simulink library "DCMotorLibrary"  (R2020a)
settings: Solver=ode45  StartTime=0.0  StopTime=10.0  RelTol=1e-3
undefined symbols (not defined in the file or in its folder): b, deg, F, Fs, J, K, L, Motor, Motor_Lib, NULL, R, s, serial
libraries: fl_lib x69, nesl_utility x46, mblibv1 x13, ee_lib x12, sdl_lib x3, sm_lib x3, instrumentlib x3, simulink_extras x3, speedgoatlib_IO101 x3, simulink x1, $bdroot x1, demoLibrary x1
(part 1 of 2)
settings Model: Creator=deastman  LastModifiedBy=RAJENDRA PHUTANE
settings DataIOCC: LimitDataPoints=on  SaveFormat=Array  ReturnWorkspaceOutputs=off
settings OptimizationCC: BlockReduction=off  BooleanDataType=off  LifeSpan=inf
settings DebuggingCC: SaveWithParameterizedLinksMsg=none  UnderspecifiedInitializationDetection=Classic  MergeDetectMultiDrivingBlocksExec=none  SignalResolutionControl=TryResolveAllWithWarning  SFUnexpectedBacktrackingDiag=warning  SFNoUnconditionalDefaultTransitionDiag=warning  SFExecutionAtInitializationDiag=none  ArithmeticOperatorsInVariantConditions=warning
settings HardwareCC: ProdBitPerPointer=32  ProdBitPerSizeT=32  ProdBitPerPtrDiffT=32  ProdLargestAtomicFloat=None  ProdIntDivRoundTo=Undefined  ProdEndianess=Unspecified  ProdWordSize=32  ProdHWDeviceType=32-bit Generic  TargetUnknown=on
settings ModelReferenceCC: PropagateSignalLabelsOutOfModel=off
settings SFSimCC: SimUseLocalCustomCode=off  CustomCodeUndefinedFunction=UseInterfaceOnly
settings RTWCC: RTWUseLocalCustomCode=off
settings CodeAppCC: StateflowObjectComments=on
settings GRTTargetCC: TargetLangStandard=C89/C90 (ANSI)
settings ConfigComp: CovMetricSettings=dw  CovHtmlReporting=on  CovSaveCumulativeToWorkspaceVar=on  CovSaveSingleToWorkspaceVar=on  CovExternalEMLEnable=off  CovSFcnEnable=off

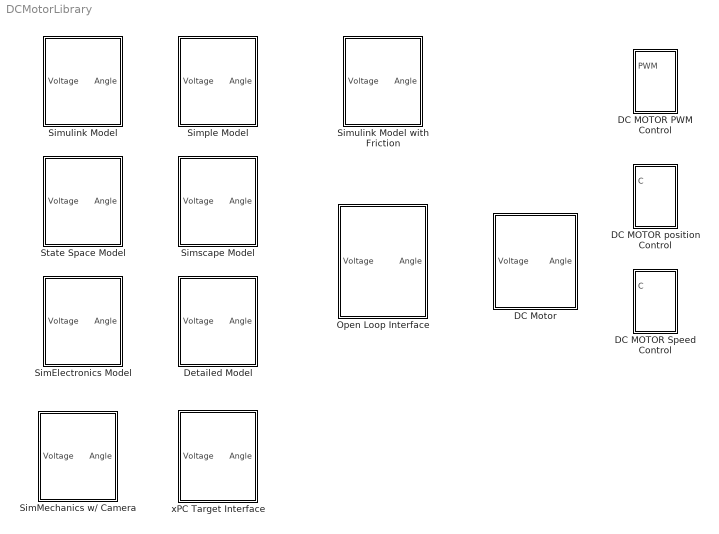
== system DCMotorLibrary ==
  DC MOTOR PWM Control : Subsystem
  DC MOTOR Speed Control : Subsystem
  DC MOTOR position Control : Subsystem
  DC Motor : Subsystem  BlockChoice=Open Loop Interface
      settings: TemplateBlock=self  MemberBlocks=Detailed Model,Open Loop Interface,SimElectronics Model,SimMechanics w/ Camera,Simple Model,Simscape Model,Simulink Model,Simulink Model with Friction,State Space Model,xPC Target Interface
  Detailed Model : Subsystem  mask(DC Motor){b=b, J=J, F=F, Fs=Fs, voltGain=1, Td=0.01}
      mask prompts: b "Damping Coefficient:"; J "Rotor Inertia:"; F "Friction:"; Fs "Staic Friction Gain:"; voltGain "Amplifier Gain:"; Td "Measurement Delay:"
      mask help:
      | This block simulates a basic brushed DC Motor with voltage input and rotor
      | angle in degrees as the output.
      mask Display: image(imread('dcmotor.jpg'))
  Open Loop Interface : Subsystem
      mask Display: image(imread('hs422.jpg'))
  SimElectronics Model : Subsystem  mask(DC Motor){K=K, R=R, L=L, b=b, J=J}
      mask prompts: K "Torque Constant:"; R "Armature Resistance:"; L "Armature Inductance:"; b "Damping Coefficient:"; J "Rotor Inertia:"
      mask help:
      | This block simulates a basic brushed DC Motor with voltage input and rotor
      | angle in degrees as the output.
      mask Display: image(imread('dcmotor.jpg'))
  SimMechanics w/ Camera : Subsystem  mask(DC Motor){K=K, R=R, L=L, b=b, J=J, Td=0.01}
      mask prompts: K "Torque Constant [N*m/A]"; R "Armature Resistance [Ohm]"; L "Armature Inductance [H]"; b "Damping Coefficient [N*m/(rad/s)]"; J "Rotor Inertia [g*cm^2]"; Td "Measurement Delay [s]"
      mask help:
      | This block simulates a basic brushed DC Motor with voltage input and rotor
      | angle in degrees as the output.
      mask Display: image(imread('dcmotor.jpg'))
  Simple Model : Subsystem  mask(DC Motor){K=K, F=F, Td=0}
      mask prompts: K "Motor Gain:"; F "Friction:"; Td "Time Delay:"
      mask help:
      | This block simulates a basic brushed DC Motor with voltage input and rotor
      | angle in degrees as the output.
      mask Display: image(imread('dcmotor.jpg'))
  Simscape Model : Subsystem  mask(DC Motor){K=K, R=R, L=L, b=b, J=J}
      mask prompts: K "Torque Constant:"; R "Armature Resistance:"; L "Armature Inductance:"; b "Damping Coefficient:"; J "Rotor Inertia:"
      mask help:
      | This block simulates a basic brushed DC Motor with voltage input and rotor
      | angle in degrees as the output.
      mask Display: image(imread('dcmotor.jpg'))
  Simulink Model : Subsystem  mask(DC Motor){K=K, R=R, L=L, b=b, J=J}
      mask prompts: K "Torque Constant:"; R "Armature Resistance:"; L "Armature Inductance:"; b "Damping Coefficient:"; J "Rotor Inertia:"
      mask help:
      | This block simulates a basic brushed DC Motor with voltage input and rotor
      | angle in degrees as the output.
      mask Display: image(imread('dcmotor.jpg'))
  Simulink Model with Friction : Subsystem  AncestorBlock=demoLibrary/Motor Models/Simulink Model  mask(DC Motor){K=K, R=R, L=L, F=F, Fs=Fs, J=J}
      mask prompts: K "Torque Constant:"; R "Armature Resistance:"; L "Armature Inductance:"; F "Coulomb Friction Torque:"; Fs "Static Friction Torque"; J "Rotor Inertia:"
      mask help:
      | This block simulates a basic brushed DC Motor with voltage input and rotor
      | angle in degrees as the output.
      mask Display: image(imread('dcmotor.jpg'))
  State Space Model : Subsystem  mask(DC Motor){K=K, R=R, L=L, b=b, J=J}
      mask prompts: K "Torque Constant:"; R "Armature Resistance:"; L "Armature Inductance:"; b "Damping Coefficient:"; J "Rotor Inertia:"
      mask help:
      | This block simulates a basic brushed DC Motor with voltage input and rotor
      | angle in degrees as the output.
      mask Display: image(imread('dcmotor.jpg'))
  xPC Target Interface : Subsystem
      mask Display: image(imread('xPCTargetDCMotor.jpg'))

== system DCMotorLibrary/DC MOTOR PWM Control ==
  PWM : Inport
  DC Source : fl_lib/Electrical/Electrical Sources/DC Voltage Source  v0=12 V
  ERef : fl_lib/Electrical/Electrical Elements/Electrical Reference
  Motor1 : Subsystem  VariantControl=Motor
      mask Display: image('youBot_Arm_Actuation_Motor_Motor_IMAGE.jpg');
  Scope : Scope
  Solver Configuration : nesl_utility/Solver Configuration  PhysicalDomain=network_engine_domain  SubClassName=solver  LeftPortType=input  RightPortType=generic  Tones=[]  Harmonics=[]  SimulateNoise=off  Profile=off  UseLocalSampling=off  EnableSwitchedLinearOptims=on  FrequencyDomain=off  UseCCode=off  RelTol=0.001  AbsTol=1e-06  MinStep=1e-09  ToWorkspace=off  RevertToSquareIcSolve=off  NumHomotopyIterations=100  PhasorMode=off  PhasorModeNumHarmonics=1  DoDC=off  ResidualTolerance=1e-09  UseLocalSolver=off  LocalSolverChoice=NE_BACKWARD_EULER_ADVANCER  LocalSolverSampleTime=0.001  DoFixedCost=off  MaxNonlinIter=3  MaxModeIter=2  LinearAlgebra=auto  EquationFormulation=NE_TIME_EF  DelaysMemoryBudget=1024  AutomaticFiltering=on  FilteringTimeConstant=0.001  PartitionStorageMethod=AS_NEEDED  PartitionMemoryBudget=1024  PartitionMethod=ROBUST
  F : PMIOPort  Side=Right
  B : PMIOPort  Port=2  Side=Left
  wires:
  Motor1/1(m) -> Scope/1
  PWM/1 -> Motor1/1(PWM)
  connections:
  DC Source/RConn1 -- Motor1/RConn2 -- ERef/LConn1
  DC Source/LConn1 -- Motor1/LConn2 -- Solver Configuration/RConn1
  Motor1/LConn1 -- B/RConn1
  Motor1/RConn1 -- F/RConn1

== system DCMotorLibrary/DC MOTOR Speed Control ==
  C : Inport
  DC Source : fl_lib/Electrical/Electrical Sources/DC Voltage Source  v0=12 V
  ERef : fl_lib/Electrical/Electrical Elements/Electrical Reference
  Motor1 : Subsystem  VariantControl=Motor
      mask Display: image('youBot_Arm_Actuation_Motor_Motor_IMAGE.jpg');
  Solver Configuration : nesl_utility/Solver Configuration  PhysicalDomain=network_engine_domain  SubClassName=solver  LeftPortType=input  RightPortType=generic  Tones=[]  Harmonics=[]  SimulateNoise=off  Profile=off  UseLocalSampling=off  EnableSwitchedLinearOptims=on  FrequencyDomain=off  UseCCode=off  RelTol=0.001  AbsTol=1e-06  MinStep=1e-09  ToWorkspace=off  RevertToSquareIcSolve=off  NumHomotopyIterations=100  PhasorMode=off  PhasorModeNumHarmonics=1  DoDC=off  ResidualTolerance=1e-09  UseLocalSolver=off  LocalSolverChoice=NE_BACKWARD_EULER_ADVANCER  LocalSolverSampleTime=0.001  DoFixedCost=off  MaxNonlinIter=3  MaxModeIter=2  LinearAlgebra=auto  EquationFormulation=NE_TIME_EF  DelaysMemoryBudget=1024  AutomaticFiltering=on  FilteringTimeConstant=0.001  PartitionStorageMethod=AS_NEEDED  PartitionMemoryBudget=1024  PartitionMethod=ROBUST
  Terminator : Terminator
  F : PMIOPort  Side=Right
  B : PMIOPort  Port=2  Side=Left
  wires:
  Motor1/1(m) -> Terminator/1
  C/1 -> Motor1/1(C)
  connections:
  DC Source/RConn1 -- Motor1/RConn2 -- ERef/LConn1
  DC Source/LConn1 -- Motor1/LConn2 -- Solver Configuration/RConn1
  Motor1/LConn1 -- B/RConn1
  Motor1/RConn1 -- F/RConn1

== system DCMotorLibrary/DC MOTOR position Control ==
  C : Inport
  DC Source : fl_lib/Electrical/Electrical Sources/DC Voltage Source  v0=12 V
  ERef : fl_lib/Electrical/Electrical Elements/Electrical Reference
  Motor1 : Subsystem  VariantControl=Motor
      mask Display: image('youBot_Arm_Actuation_Motor_Motor_IMAGE.jpg');
  Solver Configuration : nesl_utility/Solver Configuration  PhysicalDomain=network_engine_domain  SubClassName=solver  LeftPortType=input  RightPortType=generic  Tones=[]  Harmonics=[]  SimulateNoise=off  Profile=off  UseLocalSampling=off  EnableSwitchedLinearOptims=on  FrequencyDomain=off  UseCCode=off  RelTol=0.001  AbsTol=1e-06  MinStep=1e-09  ToWorkspace=off  RevertToSquareIcSolve=off  NumHomotopyIterations=100  PhasorMode=off  PhasorModeNumHarmonics=1  DoDC=off  ResidualTolerance=1e-09  UseLocalSolver=off  LocalSolverChoice=NE_BACKWARD_EULER_ADVANCER  LocalSolverSampleTime=0.001  DoFixedCost=off  MaxNonlinIter=3  MaxModeIter=2  LinearAlgebra=auto  EquationFormulation=NE_TIME_EF  DelaysMemoryBudget=1024  AutomaticFiltering=on  FilteringTimeConstant=0.001  PartitionStorageMethod=AS_NEEDED  PartitionMemoryBudget=1024  PartitionMethod=ROBUST
  Terminator : Terminator
  F : PMIOPort  Side=Right
  B : PMIOPort  Port=2  Side=Left
  wires:
  C/1 -> Motor1/1(C)
  Motor1/1(m) -> Terminator/1
  connections:
  Motor1/RConn1 -- F/RConn1
  Motor1/LConn1 -- B/RConn1
  Solver Configuration/RConn1 -- Motor1/LConn2 -- DC Source/LConn1
  ERef/LConn1 -- Motor1/RConn2 -- DC Source/RConn1

== system DCMotorLibrary/DC Motor ==
  Voltage : Inport
  Open Loop Interface : $bdroot/Motor Models/Open Loop Interface  SystemSampleTime=-1  Latency=0  AutoFrameSizeCalculation=off
  Angle : Outport
  wires:
  Voltage/1 -> Open Loop Interface/1
  Open Loop Interface/1 -> Angle/1

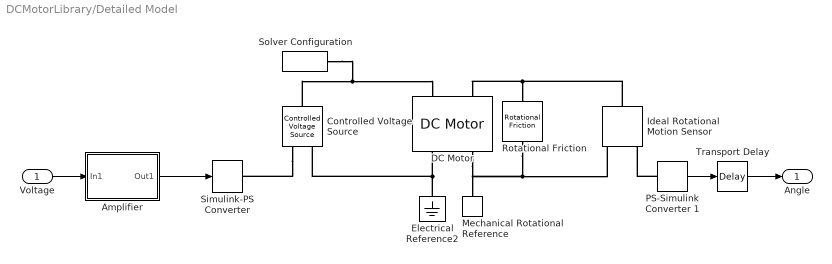
== system DCMotorLibrary/Detailed Model ==
  Voltage : Inport
  Amplifier : Subsystem
  Controlled Voltage Source : fl_lib/Electrical/Electrical Sources/Controlled Voltage Source
  DC Motor : ee_lib/Electromechanical/Brushed Motors/DC Motor  field_option=ee.enum.field_option.pm  Rf=100 Ohm  Lf=1 H  Laf=0.15 H  If0=0 A  parameterization=2  Ra=8 Ohm  La=1.5e-3 H  emf_or_torque=1  Kv=1 V/(rad/s)  Ki=6.876e-04 N*m/A  T_stall=57/16 in*lbf  w_max=62.5 rpm  w_rated=1.5e+04 rpm  P_rated=0.08 W  V_rated=5 V  J=J kg*m^2  lam_param=1  lam=b N*m/(rad/s)  i_noload=0 A  V_i_noload=1.5 V  speed0=0 rpm  alpha=3.93e-3 1/K  Tmeas=25 degC  thermal_mass=100 J/K  initial_temperature=25 degC
  Electrical Reference2 : fl_lib/Electrical/Electrical Elements/Electrical Reference
  Ideal Rotational Motion Sensor : fl_lib/Mechanical/Mechanical Sensors/Ideal Rotational Motion Sensor  wrap_angle=simscape.enum.onoff.off  offset=0 rad
  Mechanical Rotational Reference : fl_lib/Mechanical/Rotational Elements/Mechanical Rotational Reference
  PS-Simulink Converter 1 : nesl_utility/PS-Simulink Converter  PhysicalDomain=network_engine_domain  SubClassName=ps_output  LeftPortType=input  RightPortType=output  PseudoPeriodic=off  Frequencies=[]  Unit=deg  AffineConversion=off
  Rotational Friction : fl_lib/Mechanical/Rotational Elements/Rotational Friction  brkwy_trq=F*Fs N*m  brkwy_vel=0.060623 rad/s  Col_trq=F N*m  visc_coef=0.001 N*m/(rad/s)  w_specify=off  w_priority=High  w=0 rad/s  w_nominal_specify=off  w_nominal_unit=rad/s  w_nominal_value=1  t_specify=off  t_priority=High  t=0 N*m  t_nominal_specify=off  t_nominal_unit=N*m  t_nominal_value=1
  Simulink-PS Converter : nesl_utility/Simulink-PS Converter  PhysicalDomain=network_engine_domain  SubClassName=ps_input  LeftPortType=input  RightPortType=output  PseudoPeriodic=off  Frequencies=[]  NoiseDistribution=none  NoiseParameters=[]  Unit=1  AffineConversion=off  FilteringAndDerivatives=zero  SimscapeFilterOrder=1  InputFilterTimeConstant=.001  UdotUserProvided=0
  Solver Configuration : nesl_utility/Solver Configuration  PhysicalDomain=network_engine_domain  SubClassName=solver  LeftPortType=input  RightPortType=generic  Tones=[]  Harmonics=[]  SimulateNoise=off  Profile=off  UseLocalSampling=off  EnableSwitchedLinearOptims=on  FrequencyDomain=off  UseCCode=off  RelTol=0.001  AbsTol=1e-06  MinStep=1e-09  ToWorkspace=off  RevertToSquareIcSolve=off  NumHomotopyIterations=100  PhasorMode=off  PhasorModeNumHarmonics=1  DoDC=off  ResidualTolerance=1e-9  UseLocalSolver=off  LocalSolverChoice=NE_BACKWARD_EULER_ADVANCER  LocalSolverSampleTime=.001  DoFixedCost=off  MaxNonlinIter=12  MaxModeIter=2  LinearAlgebra=Sparse  EquationFormulation=NE_TIME_EF  DelaysMemoryBudget=1024  AutomaticFiltering=on  FilteringTimeConstant=0.001  PartitionStorageMethod=AS_NEEDED  PartitionMemoryBudget=1024  PartitionMethod=FAST
  Transport Delay : TransportDelay  DelayTime=Td  PadeOrder=4
  Angle : Outport
  wires:
  Voltage/1 -> Amplifier/1(In1)
  PS-Simulink Converter 1/1 -> Transport Delay/1
  Transport Delay/1 -> Angle/1
  Amplifier/1(Out1) -> Simulink-PS Converter/1
  connections:
  Ideal Rotational Motion Sensor/LConn1 -- DC Motor/LConn2 -- Rotational Friction/LConn1
  Controlled Voltage Source/RConn1 -- Simulink-PS Converter/RConn1
  PS-Simulink Converter 1/LConn1 -- Ideal Rotational Motion Sensor/RConn3
  Mechanical Rotational Reference/LConn1 -- DC Motor/RConn2 -- Ideal Rotational Motion Sensor/RConn1 -- Rotational Friction/RConn1
  Controlled Voltage Source/LConn1 -- DC Motor/LConn1 -- Solver Configuration/RConn1
  Electrical Reference2/LConn1 -- DC Motor/RConn1 -- Controlled Voltage Source/RConn2

== system DCMotorLibrary/Open Loop Interface ==
  Voltage : Inport
  Bias : Bias  Bias=5
  Gain : Gain  Gain=255/10  OutDataTypeStr=uint8
  Saturation1 : Saturate  UpperLimit=5  LowerLimit=-5
  Serial Motor Interface : Subsystem  AncestorBlock=demoLibrary/Utilities/Serial Motor Interface
  Simulation Pace : aerolibanimutils/Simulation Pace  SimulationPace=1  SleepMode=MATLAB Thread  OutputPaceError=off  SampleTime=1/50
      settings: AttributesFormatString=%<SimulationPace> sec/sec
  Angle : Outport  PortDimensions=1
  wires:
  Voltage/1 -> Saturation1/1
  Serial Motor Interface/1(Angle) -> Angle/1
  Saturation1/1 -> Bias/1
  Bias/1 -> Gain/1
  Gain/1 -> Serial Motor Interface/1(command)

== system DCMotorLibrary/SimElectronics Model ==
  Voltage : Inport
  Controlled Voltage Source : fl_lib/Electrical/Electrical Sources/Controlled Voltage Source
  DC Motor : ee_lib/Electromechanical/Brushed Motors/DC Motor  field_option=ee.enum.field_option.pm  Rf=100 Ohm  Lf=1 H  Laf=0.15 H  If0=0 A  parameterization=1  Ra=R Ohm  La=L H  emf_or_torque=1  Kv=K V/(rad/s)  Ki=6.876e-04 N*m/A  T_stall=2.4e-04 N*m  w_max=1.91e+04 rpm  w_rated=1.5e+04 rpm  P_rated=0.08 W  V_rated=1.5 V  J=J kg*m^2  lam_param=1  lam=b N*m/(rad/s)  i_noload=0 A  V_i_noload=1.5 V  speed0=0 rpm  alpha=3.93e-3 1/K  Tmeas=25 degC  thermal_mass=100 J/K  initial_temperature=25 degC
  Electrical Reference2 : fl_lib/Electrical/Electrical Elements/Electrical Reference
  Ideal Rotational Motion Sensor : fl_lib/Mechanical/Mechanical Sensors/Ideal Rotational Motion Sensor  wrap_angle=simscape.enum.onoff.off  offset=0 rad
  Mechanical Rotational Reference : fl_lib/Mechanical/Rotational Elements/Mechanical Rotational Reference
  PS-Simulink Converter 1 : nesl_utility/PS-Simulink Converter  PhysicalDomain=network_engine_domain  SubClassName=ps_output  LeftPortType=input  RightPortType=output  PseudoPeriodic=off  Frequencies=[]  Unit=deg  AffineConversion=off
  Simulink-PS Converter : nesl_utility/Simulink-PS Converter  PhysicalDomain=network_engine_domain  SubClassName=ps_input  LeftPortType=input  RightPortType=output  PseudoPeriodic=off  Frequencies=[]  NoiseDistribution=none  NoiseParameters=[]  Unit=1  AffineConversion=off  FilteringAndDerivatives=zero  SimscapeFilterOrder=1  InputFilterTimeConstant=.001  UdotUserProvided=0
  Solver Configuration : nesl_utility/Solver Configuration  PhysicalDomain=network_engine_domain  SubClassName=solver  LeftPortType=input  RightPortType=generic  Tones=[]  Harmonics=[]  SimulateNoise=off  Profile=off  UseLocalSampling=off  EnableSwitchedLinearOptims=on  FrequencyDomain=off  UseCCode=off  RelTol=0.001  AbsTol=1e-06  MinStep=1e-09  ToWorkspace=off  RevertToSquareIcSolve=off  NumHomotopyIterations=100  PhasorMode=off  PhasorModeNumHarmonics=1  DoDC=off  ResidualTolerance=1e-9  UseLocalSolver=off  LocalSolverChoice=NE_BACKWARD_EULER_ADVANCER  LocalSolverSampleTime=.001  DoFixedCost=off  MaxNonlinIter=3  MaxModeIter=2  LinearAlgebra=Sparse  EquationFormulation=NE_TIME_EF  DelaysMemoryBudget=1024  AutomaticFiltering=on  FilteringTimeConstant=0.001  PartitionStorageMethod=AS_NEEDED  PartitionMemoryBudget=1024  PartitionMethod=FAST
  Angle : Outport
  wires:
  PS-Simulink Converter 1/1 -> Angle/1
  Voltage/1 -> Simulink-PS Converter/1
  connections:
  DC Motor/LConn1 -- Solver Configuration/RConn1 -- Controlled Voltage Source/LConn1
  DC Motor/RConn1 -- Controlled Voltage Source/RConn2 -- Electrical Reference2/LConn1
  DC Motor/RConn2 -- Ideal Rotational Motion Sensor/RConn1 -- Mechanical Rotational Reference/LConn1
  PS-Simulink Converter 1/LConn1 -- Ideal Rotational Motion Sensor/RConn3
  Controlled Voltage Source/RConn1 -- Simulink-PS Converter/RConn1
  Ideal Rotational Motion Sensor/LConn1 -- DC Motor/LConn2

== system DCMotorLibrary/SimMechanics w// Camera ==
  Voltage : Inport
  Controlled Voltage Source : fl_lib/Electrical/Electrical Sources/Controlled Voltage Source
  DC Motor : ee_lib/Electromechanical/Brushed Motors/DC Motor  field_option=ee.enum.field_option.pm  Rf=100 Ohm  Lf=1 H  Laf=0.15 H  If0=0 A  parameterization=1  Ra=R Ohm  La=L H  emf_or_torque=2  Kv=7.2e-05 V/rpm  Ki=K N*m/A  T_stall=2.4e-04 N*m  w_max=1.91e+04 rpm  w_rated=1.5e+04 rpm  P_rated=0.08 W  V_rated=1.5 V  J=J g*cm^2  lam_param=1  lam=b N*m/(rad/s)  i_noload=0 A  V_i_noload=1.5 V  speed0=0 rpm  alpha=3.93e-3 1/K  Tmeas=25 degC  thermal_mass=100 J/K  initial_temperature=25 degC
  Electrical Reference : fl_lib/Electrical/Electrical Elements/Electrical Reference
  Mechanical Rotational Reference : fl_lib/Mechanical/Rotational Elements/Mechanical Rotational Reference
  Mechanical part : Subsystem
      mask Display: image(imread('hs422.jpg'))
  Revolute - Rotational Interface : mblibv1/Interface  Elements/Revolute - Rotational Interface  UpdateFromCAD=off  DialogClass=RevoluteRotationalInterface  Primitive=R1  InputFiltering=off  SimscapeFilterOrder=1  InputFilterTimeConstant=0.001
  Simulink-PS Converter : nesl_utility/Simulink-PS Converter  PhysicalDomain=network_engine_domain  SubClassName=ps_input  LeftPortType=input  RightPortType=output  PseudoPeriodic=off  Frequencies=[]  NoiseDistribution=none  NoiseParameters=[]  Unit=1  AffineConversion=off  FilteringAndDerivatives=filter  SimscapeFilterOrder=2  InputFilterTimeConstant=.001  UdotUserProvided=1
  Solver Configuration : nesl_utility/Solver Configuration  PhysicalDomain=network_engine_domain  SubClassName=solver  LeftPortType=input  RightPortType=generic  Tones=[]  Harmonics=[]  SimulateNoise=off  Profile=off  UseLocalSampling=off  EnableSwitchedLinearOptims=on  FrequencyDomain=off  UseCCode=off  RelTol=0.001  AbsTol=1e-06  MinStep=1e-09  ToWorkspace=off  RevertToSquareIcSolve=off  NumHomotopyIterations=100  PhasorMode=off  PhasorModeNumHarmonics=1  DoDC=off  ResidualTolerance=1e-9  UseLocalSolver=on  LocalSolverChoice=NE_BACKWARD_EULER_ADVANCER  LocalSolverSampleTime=.001  DoFixedCost=off  MaxNonlinIter=12  MaxModeIter=2  LinearAlgebra=Sparse  EquationFormulation=NE_TIME_EF  DelaysMemoryBudget=1024  AutomaticFiltering=on  FilteringTimeConstant=0.001  PartitionStorageMethod=AS_NEEDED  PartitionMemoryBudget=1024  PartitionMethod=FAST
  Transport Delay : TransportDelay  DelayTime=Td  PadeOrder=4
  Angle : Outport
  wires:
  Transport Delay/1 -> Angle/1
  Mechanical part/1(Angle) -> Transport Delay/1
  Voltage/1 -> Simulink-PS Converter/1
  connections:
  Revolute - Rotational Interface/RConn1 -- Mechanical part/LConn1
  DC Motor/LConn2 -- Revolute - Rotational Interface/LConn1
  Simulink-PS Converter/RConn1 -- Controlled Voltage Source/RConn1
  Mechanical Rotational Reference/LConn1 -- Revolute - Rotational Interface/LConn2 -- DC Motor/RConn2
  Solver Configuration/RConn1 -- Controlled Voltage Source/LConn1 -- DC Motor/LConn1
  Controlled Voltage Source/RConn2 -- DC Motor/RConn1 -- Electrical Reference/LConn1

== system DCMotorLibrary/Simple Model ==
  Voltage : Inport
  Dead Zone : DeadZone  LowerValue=-F  UpperValue=F  SaturateOnIntegerOverflow=on
  Gain : Gain  Gain=K
  Integrator : Integrator
  Transport Delay : TransportDelay  DelayTime=Td  PadeOrder=4
  Angle : Outport
  wires:
  Dead Zone/1 -> Gain/1
  Voltage/1 -> Dead Zone/1
  Integrator/1 -> Transport Delay/1
  Gain/1 -> Integrator/1
  Transport Delay/1 -> Angle/1

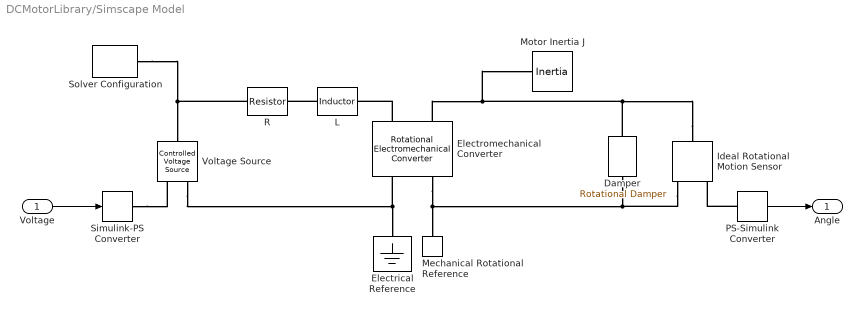
== system DCMotorLibrary/Simscape Model ==
  Voltage : Inport
  Damper : fl_lib/Mechanical/Rotational Elements/Rotational Damper  D=b N*m/(rad/s)  w_specify=off  w_priority=None  w=0 rad/s  w_nominal_specify=off  w_nominal_unit=rad/s  w_nominal_value=1  t_specify=off  t_priority=None  t=0 N*m  t_nominal_specify=off  t_nominal_unit=N*m  t_nominal_value=1
  Electrical Reference : fl_lib/Electrical/Electrical Elements/Electrical Reference
  Electromechanical Converter : fl_lib/Electrical/Electrical Elements/Rotational Electromechanical Converter  K=K V/(rad/s)  i_specify=off  i_priority=None  i=0 A  i_nominal_specify=off  i_nominal_unit=A  i_nominal_value=1  v_specify=off  v_priority=None  v=0 V  v_nominal_specify=off  v_nominal_unit=V  v_nominal_value=1  t_specify=off  t_priority=None  t=0 N*m  t_nominal_specify=off  t_nominal_unit=N*m  t_nominal_value=1  w_specify=off  w_priority=None  w=0 rad/s  w_nominal_specify=off  w_nominal_unit=rad/s  w_nominal_value=1
  Ideal Rotational Motion Sensor : fl_lib/Mechanical/Mechanical Sensors/Ideal Rotational Motion Sensor  wrap_angle=simscape.enum.onoff.off  offset=0 deg
  L : fl_lib/Electrical/Electrical Elements/Inductor  l=L H  r=0 Ohm  g=1e-09 1/Ohm  i_specify=off  i_priority=None  i=0 A  i_nominal_specify=off  i_nominal_unit=A  i_nominal_value=1  v_specify=off  v_priority=None  v=0 V  v_nominal_specify=off  v_nominal_unit=V  v_nominal_value=1  i_L_specify=on  i_L_priority=High  i_L=0 A  i_L_nominal_specify=off  i_L_nominal_unit=A  i_L_nominal_value=1
  Mechanical Rotational Reference : fl_lib/Mechanical/Rotational Elements/Mechanical Rotational Reference
  Motor Inertia J : fl_lib/Mechanical/Rotational Elements/Inertia  inertia=J kg*m^2  w_specify=on  w_priority=High  w=0 rad/s  w_nominal_specify=off  w_nominal_unit=rad/s  w_nominal_value=1  t_specify=off  t_priority=None  t=0 N*m  t_nominal_specify=off  t_nominal_unit=N*m  t_nominal_value=1
  PS-Simulink Converter : nesl_utility/PS-Simulink Converter  PhysicalDomain=network_engine_domain  SubClassName=ps_output  LeftPortType=input  RightPortType=output  PseudoPeriodic=off  Frequencies=[]  Unit=deg  AffineConversion=off
  R : fl_lib/Electrical/Electrical Elements/Resistor  Tag=Factory Generic  R=R Ohm  i_specify=off  i_priority=None  i=0 A  i_nominal_specify=off  i_nominal_unit=A  i_nominal_value=1  v_specify=off  v_priority=None  v=0 V  v_nominal_specify=off  v_nominal_unit=V  v_nominal_value=1
  Simulink-PS Converter : nesl_utility/Simulink-PS Converter  PhysicalDomain=network_engine_domain  SubClassName=ps_input  LeftPortType=input  RightPortType=output  PseudoPeriodic=off  Frequencies=[]  NoiseDistribution=none  NoiseParameters=[]  Unit=V  AffineConversion=off  FilteringAndDerivatives=zero  SimscapeFilterOrder=1  InputFilterTimeConstant=.001  UdotUserProvided=0
  Solver Configuration : nesl_utility/Solver Configuration  PhysicalDomain=network_engine_domain  SubClassName=solver  LeftPortType=input  RightPortType=generic  Tones=[]  Harmonics=[]  SimulateNoise=off  Profile=off  UseLocalSampling=off  EnableSwitchedLinearOptims=on  FrequencyDomain=off  UseCCode=off  RelTol=0.001  AbsTol=1e-06  MinStep=1e-09  ToWorkspace=off  RevertToSquareIcSolve=off  NumHomotopyIterations=100  PhasorMode=off  PhasorModeNumHarmonics=1  DoDC=off  ResidualTolerance=1e-9  UseLocalSolver=off  LocalSolverChoice=NE_BACKWARD_EULER_ADVANCER  LocalSolverSampleTime=.001  DoFixedCost=off  MaxNonlinIter=3  MaxModeIter=2  LinearAlgebra=Sparse  EquationFormulation=NE_TIME_EF  DelaysMemoryBudget=1024  AutomaticFiltering=on  FilteringTimeConstant=0.001  PartitionStorageMethod=AS_NEEDED  PartitionMemoryBudget=1024  PartitionMethod=FAST
  Voltage Source : fl_lib/Electrical/Electrical Sources/Controlled Voltage Source
  Angle : Outport
  wires:
  Voltage/1 -> Simulink-PS Converter/1
  PS-Simulink Converter/1 -> Angle/1
  connections:
  R/LConn1 -- Solver Configuration/RConn1 -- Voltage Source/LConn1
  Electromechanical Converter/RConn1 -- Voltage Source/RConn2 -- Electrical Reference/LConn1
  Ideal Rotational Motion Sensor/LConn1 -- Electromechanical Converter/LConn2 -- Motor Inertia J/LConn1 -- Damper/LConn1
  Ideal Rotational Motion Sensor/RConn1 -- Damper/RConn1 -- Mechanical Rotational Reference/LConn1 -- Electromechanical Converter/RConn2
  Simulink-PS Converter/RConn1 -- Voltage Source/RConn1
  Electromechanical Converter/LConn1 -- L/RConn1
  L/LConn1 -- R/RConn1
  PS-Simulink Converter/LConn1 -- Ideal Rotational Motion Sensor/RConn3

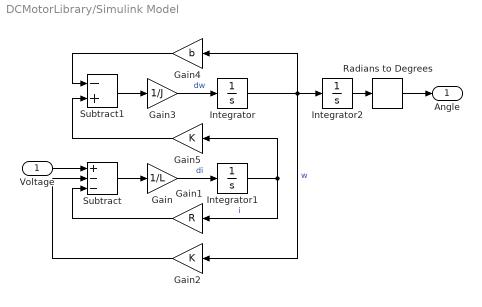
== system DCMotorLibrary/Simulink Model ==
  Voltage : Inport
  Gain : Gain  Gain=1/L
  Gain1 : Gain  Gain=R
  Gain2 : Gain  Gain=K
  Gain3 : Gain  Gain=1/J
  Gain4 : Gain  Gain=b
  Gain5 : Gain  Gain=K
  Integrator : Integrator
  Integrator1 : Integrator
  Integrator2 : Integrator
  Radians to Degrees : simulink_extras/Transformations/Radians to Degrees
  Subtract : Sum  Inputs=+--
  Subtract1 : Sum  Inputs=-+
  Angle : Outport
  wires:
  Voltage/1 -> Subtract/1
  Integrator2/1 -> Radians to Degrees/1
  Gain5/1 -> Subtract1/2
  Gain4/1 -> Subtract1/1
  Subtract1/1 -> Gain3/1
  Gain2/1 -> Subtract/2
  Gain1/1 -> Subtract/3
  Subtract/1 -> Gain/1
  Integrator1/1 -> Gain1/1, Gain5/1  "i"
  Integrator/1 -> Integrator2/1, Gain2/1, Gain4/1  "w"
  Gain/1 -> Integrator1/1  "di"
  Gain3/1 -> Integrator/1  "dw"
  Radians to Degrees/1 -> Angle/1

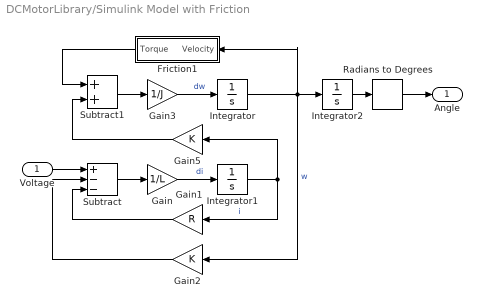
== system DCMotorLibrary/Simulink Model with Friction ==
  Voltage : Inport
  Friction1 : Subsystem  mask{FrictionStatic=Fs, FrictionCoulomb=F, eps=0.005}
      mask prompts: FrictionStatic "Static Friction Torque (Nm)"; FrictionCoulomb "Coulomb Friction Torque (Nm)"; eps "Epsilon (deg/s)"
  Gain : Gain  Gain=1/L
  Gain1 : Gain  Gain=R
  Gain2 : Gain  Gain=K
  Gain3 : Gain  Gain=1/J
  Gain5 : Gain  Gain=K
  Integrator : Integrator
  Integrator1 : Integrator
  Integrator2 : Integrator
  Radians to Degrees : simulink_extras/Transformations/Radians to Degrees
  Subtract : Sum  Inputs=+--
  Subtract1 : Sum
  Angle : Outport
  wires:
  Radians to Degrees/1 -> Angle/1
  Gain3/1 -> Integrator/1  "dw"
  Gain/1 -> Integrator1/1  "di"
  Integrator/1 -> Gain2/1, Friction1/1(Velocity), Integrator2/1  "w"
  Integrator1/1 -> Gain5/1, Gain1/1  "i"
  Subtract/1 -> Gain/1
  Gain1/1 -> Subtract/3
  Gain2/1 -> Subtract/2
  Subtract1/1 -> Gain3/1
  Gain5/1 -> Subtract1/2
  Integrator2/1 -> Radians to Degrees/1
  Voltage/1 -> Subtract/1
  Friction1/1(Torque) -> Subtract1/1

== system DCMotorLibrary/State Space Model ==
  Voltage : Inport
  Integrator2 : Integrator
  Radians to Degrees : simulink_extras/Transformations/Radians to Degrees
  State-Space : StateSpace  A=[-b/J K/J; -K/L -R/L]  B=[0; 1/L]  C=[1 0]  D=[0]  InitialCondition=0
  Angle : Outport
  wires:
  Integrator2/1 -> Radians to Degrees/1
  Voltage/1 -> State-Space/1
  State-Space/1 -> Integrator2/1
  Radians to Degrees/1 -> Angle/1

== system DCMotorLibrary/xPC Target Interface ==
  Voltage : Inport
  Analog input : speedgoatlib_IO101/Analog input  id=1  startChannel=2  numChannels=1  coupling=2  range=3  acqMode=1  outpMode=Values  ts=0.002  pciSlot=-1
  Digital output : speedgoatlib_IO101/Digital output  id=1  groupChannel=Upper  lowerChannel=1  upperChannel=[1,5,6]  lowerDOReset=1  upperDOReset=[0,0,0]  lowerDOInitValues=0  upperDOInitValues=[0,0,0]  ts=0.002  pciSlot=-1
  Setup : speedgoatlib_IO101/Setup  group=Digital setup upper channel  id=1  pciSlot=-1  adStartChannel=2  adNumChannel=1  adCoupling=Single-ended  adRange="-3.3 .. 3.3V ==> Set  hardware DIP switches 2 4 6 9 to ON"  adAcqMode=Standard  daChannel=[1:8]  daReset=[1]  daInitValue=[0]  lowerChannel=1  lowerDirection=Input  lowerDIDebounce=0  lowerDOReset=[1]  lowerDOInitValues=[0]  upperChannel=[1 5 6]  upperDirection=Output  upperDIDebounce=0  upperDOReset=0  upperDOInitValues=0
  SignalConditioning : SAM_lib/SignalConditioning
  Angle : Outport
  wires:
  SignalConditioning/3 -> Digital output/3
  Analog input/1 -> SignalConditioning/2
  SignalConditioning/4 -> Angle/1  "measured angle"
  Voltage/1 -> SignalConditioning/1
  SignalConditioning/1 -> Digital output/1
  SignalConditioning/2 -> Digital output/2

== system DCMotorLibrary/DC MOTOR PWM Control/Motor1 ==
  PWM : Inport
  Meas P : Subsystem  Tag=CustomStyle
      mask Display: disp('m')
  Motor : Subsystem  AncestorBlock=Motor_Lib/Motor  VariantControl=Motor  mask{r_motor=Motor.R, l_motor=Motor.L, k_motor=Motor.K, i_motor_noLoad=Motor.no_load_i, v_supply=Motor.V, gear_ratio=Motor.gr, friction_visc=Motor.friction, ctrl_deadZone=Motor.Dead_Band}
      mask prompts: r_motor "Armature Resistance (Ohm)"; l_motor "Armature Inductance (H)"; k_motor "Torque Constant (N*(m/A))"; i_motor_noLoad "No-Load Current (A)"; v_supply "Supply Voltage (V)"; gear_ratio "Gear Ratio"; friction_visc "Viscous Friction (N*m/(rad/s))"; ctrl_deadZone "Dead Zone (deg)"
      mask DialogControl Container4 Prompt: Electrical
      mask DialogControl Container5 Prompt: Mechanical
      mask DialogControl Container6 Prompt: Control
      mask Display: image('youBot_Arm_Motor_JointIntf_IMAGE.jpg');
  RevolutePivotBicep : sm_lib/Joints/Revolute Joint  JointMode=Normal  SenseConstraintForce=on  SenseConstraintForceX=off  SenseConstraintForceY=off  SenseConstraintForceZ=off  SenseConstraintTorque=off  SenseConstraintTorqueX=off  SenseConstraintTorqueY=off  SenseConstraintTorqueZ=off  SenseTotalForce=off  SenseTotalForceX=off  SenseTotalForceY=off  SenseTotalForceZ=off  SenseTotalTorque=off  SenseTotalTorqueX=off  SenseTotalTorqueY=off  SenseTotalTorqueZ=off  CompositeWrenchDir=FollowerOnBase  CompositeWrenchFrame=BaseFrame  EquilibriumPosition=0  EquilibriumPositionUnits=rad  SpringStiffness=0  SpringStiffnessUnits=N*m/rad  DampingCoefficient=0  DampingCoefficientUnits=N*m/(rad/s)  TorqueActuationMode=InputTorque  MotionActuationMode=ComputedMotion  SensePosition=on  SenseVelocity=on  SenseAcceleration=off  SenseTorqueForce=on  SenseLowerLimitTorqueForce=off  SenseUpperLimitTorqueForce=off  LowerLimitSpecify=off  LowerLimitBound=-90  LowerLimitBoundUnits=deg  LowerLimitStiffness=1e4  LowerLimitStiffnessUnits=N*m/deg  LowerLimitDamping=10  LowerLimitDampingUnits=N*m/(deg/s)  LowerLimitTransitionRegionWidth=0.1  LowerLimitTransitionRegionWidthUnits=deg  UpperLimitSpecify=off  UpperLimitBound=90  UpperLimitBoundUnits=deg  UpperLimitStiffness=1e4  UpperLimitStiffnessUnits=N*m/deg  UpperLimitDamping=10  UpperLimitDampingUnits=N*m/(deg/s)  UpperLimitTransitionRegionWidth=0.1  UpperLimitTransitionRegionWidthUnits=deg  PositionTargetSpecify=on  PositionTargetPriority=Low  PositionTargetValue=0  PositionTargetValueUnits=deg  VelocityTargetSpecify=off  VelocityTargetPriority=High  VelocityTargetValue=0  VelocityTargetValueUnits=deg/s
  Sensing i : Subsystem
      mask Display: disp('i')
  B : PMIOPort  Side=Left
  F : PMIOPort  Port=2  Side=Right
  - : PMIOPort  Port=3  Side=Right
  + : PMIOPort  Port=4  Side=Left
  m : Outport  VectorParamsAs1DForOutWhenUnconnected=off
  wires:
  Meas P/1(P) -> m/1
  PWM/1 -> Motor/1(PWM)
  connections:
  RevolutePivotBicep/RConn2 -- Meas P/LConn1
  Meas P/LConn3 -- RevolutePivotBicep/RConn4
  Meas P/LConn2 -- RevolutePivotBicep/RConn3 -- Motor/RConn1
  Motor/LConn1 -- RevolutePivotBicep/LConn2
  RevolutePivotBicep/RConn1 -- F/RConn1
  RevolutePivotBicep/LConn1 -- B/RConn1
  Sensing i/LConn1 -- Motor/RConn2
  Motor/LConn2 -- +/RConn1
  Sensing i/RConn2 -- -/RConn1
  Sensing i/RConn1 -- Meas P/LConn5
  RevolutePivotBicep/RConn5 -- Meas P/LConn4

== system DCMotorLibrary/DC MOTOR Speed Control/Motor1 ==
  C : Inport
  Meas P : Subsystem  Tag=CustomStyle
      mask Display: disp('m')
  Motor : Subsystem  AncestorBlock=Motor_Lib/Motor  VariantControl=Motor  mask{r_motor=Motor.R, l_motor=Motor.L, k_motor=Motor.K, i_motor_noLoad=Motor.no_load_i, v_supply=Motor.V, gear_ratio=Motor.gr, friction_visc=Motor.friction, ctrl_deadZone=Motor.Dead_Band}
      mask prompts: r_motor "Armature Resistance (Ohm)"; l_motor "Armature Inductance (H)"; k_motor "Torque Constant (N*(m/A))"; i_motor_noLoad "No-Load Current (A)"; v_supply "Supply Voltage (V)"; gear_ratio "Gear Ratio"; friction_visc "Viscous Friction (N*m/(rad/s))"; ctrl_deadZone "Dead Zone (deg)"
      mask DialogControl Container4 Prompt: Electrical
      mask DialogControl Container5 Prompt: Mechanical
      mask DialogControl Container6 Prompt: Control
      mask Display: image('youBot_Arm_Motor_JointIntf_IMAGE.jpg');
  RevolutePivotBicep : sm_lib/Joints/Revolute Joint  JointMode=Normal  SenseConstraintForce=on  SenseConstraintForceX=off  SenseConstraintForceY=off  SenseConstraintForceZ=off  SenseConstraintTorque=off  SenseConstraintTorqueX=off  SenseConstraintTorqueY=off  SenseConstraintTorqueZ=off  SenseTotalForce=off  SenseTotalForceX=off  SenseTotalForceY=off  SenseTotalForceZ=off  SenseTotalTorque=off  SenseTotalTorqueX=off  SenseTotalTorqueY=off  SenseTotalTorqueZ=off  CompositeWrenchDir=FollowerOnBase  CompositeWrenchFrame=BaseFrame  EquilibriumPosition=0  EquilibriumPositionUnits=rad  SpringStiffness=0  SpringStiffnessUnits=N*m/rad  DampingCoefficient=0  DampingCoefficientUnits=N*m/(rad/s)  TorqueActuationMode=InputTorque  MotionActuationMode=ComputedMotion  SensePosition=on  SenseVelocity=on  SenseAcceleration=off  SenseTorqueForce=on  SenseLowerLimitTorqueForce=off  SenseUpperLimitTorqueForce=off  LowerLimitSpecify=off  LowerLimitBound=-90  LowerLimitBoundUnits=deg  LowerLimitStiffness=1e4  LowerLimitStiffnessUnits=N*m/deg  LowerLimitDamping=10  LowerLimitDampingUnits=N*m/(deg/s)  LowerLimitTransitionRegionWidth=0.1  LowerLimitTransitionRegionWidthUnits=deg  UpperLimitSpecify=off  UpperLimitBound=90  UpperLimitBoundUnits=deg  UpperLimitStiffness=1e4  UpperLimitStiffnessUnits=N*m/deg  UpperLimitDamping=10  UpperLimitDampingUnits=N*m/(deg/s)  UpperLimitTransitionRegionWidth=0.1  UpperLimitTransitionRegionWidthUnits=deg  PositionTargetSpecify=on  PositionTargetPriority=Low  PositionTargetValue=0  PositionTargetValueUnits=deg  VelocityTargetSpecify=off  VelocityTargetPriority=High  VelocityTargetValue=0  VelocityTargetValueUnits=deg/s
  Sensing i : Subsystem
      mask Display: disp('i')
  B : PMIOPort  Side=Left
  F : PMIOPort  Port=2  Side=Right
  - : PMIOPort  Port=3  Side=Right
  + : PMIOPort  Port=4  Side=Left
  m : Outport  VectorParamsAs1DForOutWhenUnconnected=off
  wires:
  Meas P/1(P) -> m/1
  C/1 -> Motor/1(C)
  connections:
  RevolutePivotBicep/RConn2 -- Meas P/LConn1
  Meas P/LConn3 -- RevolutePivotBicep/RConn4
  RevolutePivotBicep/RConn3 -- Meas P/LConn2 -- Motor/RConn1
  Motor/LConn1 -- RevolutePivotBicep/LConn2
  RevolutePivotBicep/RConn1 -- F/RConn1
  RevolutePivotBicep/LConn1 -- B/RConn1
  Sensing i/LConn1 -- Motor/RConn2
  Motor/LConn2 -- +/RConn1
  Sensing i/RConn2 -- -/RConn1
  Sensing i/RConn1 -- Meas P/LConn5
  RevolutePivotBicep/RConn5 -- Meas P/LConn4

== system DCMotorLibrary/DC MOTOR position Control/Motor1 ==
  C : Inport
  Meas P : Subsystem  Tag=CustomStyle
      mask Display: disp('m')
  Motor : Subsystem  AncestorBlock=Motor_Lib/Motor  VariantControl=Motor  mask{r_motor=Motor.R, l_motor=Motor.L, k_motor=Motor.K, i_motor_noLoad=Motor.no_load_i, v_supply=Motor.V, gear_ratio=Motor.gr, friction_visc=Motor.friction, ctrl_deadZone=Motor.Dead_Band}
      mask prompts: r_motor "Armature Resistance (Ohm)"; l_motor "Armature Inductance (H)"; k_motor "Torque Constant (N*(m/A))"; i_motor_noLoad "No-Load Current (A)"; v_supply "Supply Voltage (V)"; gear_ratio "Gear Ratio"; friction_visc "Viscous Friction (N*m/(rad/s))"; ctrl_deadZone "Dead Zone (deg)"
      mask DialogControl Container4 Prompt: Electrical
      mask DialogControl Container5 Prompt: Mechanical
      mask DialogControl Container6 Prompt: Control
      mask Display: image('youBot_Arm_Motor_JointIntf_IMAGE.jpg');
  RevolutePivotBicep : sm_lib/Joints/Revolute Joint  JointMode=Normal  SenseConstraintForce=on  SenseConstraintForceX=off  SenseConstraintForceY=off  SenseConstraintForceZ=off  SenseConstraintTorque=off  SenseConstraintTorqueX=off  SenseConstraintTorqueY=off  SenseConstraintTorqueZ=off  SenseTotalForce=off  SenseTotalForceX=off  SenseTotalForceY=off  SenseTotalForceZ=off  SenseTotalTorque=off  SenseTotalTorqueX=off  SenseTotalTorqueY=off  SenseTotalTorqueZ=off  CompositeWrenchDir=FollowerOnBase  CompositeWrenchFrame=BaseFrame  EquilibriumPosition=0  EquilibriumPositionUnits=rad  SpringStiffness=0  SpringStiffnessUnits=N*m/rad  DampingCoefficient=0  DampingCoefficientUnits=N*m/(rad/s)  TorqueActuationMode=InputTorque  MotionActuationMode=ComputedMotion  SensePosition=on  SenseVelocity=on  SenseAcceleration=off  SenseTorqueForce=on  SenseLowerLimitTorqueForce=off  SenseUpperLimitTorqueForce=off  LowerLimitSpecify=off  LowerLimitBound=-90  LowerLimitBoundUnits=deg  LowerLimitStiffness=1e4  LowerLimitStiffnessUnits=N*m/deg  LowerLimitDamping=10  LowerLimitDampingUnits=N*m/(deg/s)  LowerLimitTransitionRegionWidth=0.1  LowerLimitTransitionRegionWidthUnits=deg  UpperLimitSpecify=off  UpperLimitBound=90  UpperLimitBoundUnits=deg  UpperLimitStiffness=1e4  UpperLimitStiffnessUnits=N*m/deg  UpperLimitDamping=10  UpperLimitDampingUnits=N*m/(deg/s)  UpperLimitTransitionRegionWidth=0.1  UpperLimitTransitionRegionWidthUnits=deg  PositionTargetSpecify=on  PositionTargetPriority=Low  PositionTargetValue=0  PositionTargetValueUnits=deg  VelocityTargetSpecify=off  VelocityTargetPriority=High  VelocityTargetValue=0  VelocityTargetValueUnits=deg/s
  Sensing i : Subsystem
      mask Display: disp('i')
  B : PMIOPort  Side=Left
  F : PMIOPort  Port=2  Side=Right
  - : PMIOPort  Port=3  Side=Right
  + : PMIOPort  Port=4  Side=Left
  m : Outport  VectorParamsAs1DForOutWhenUnconnected=off
  wires:
  C/1 -> Motor/1(C)
  Meas P/1(P) -> m/1
  connections:
  RevolutePivotBicep/RConn5 -- Meas P/LConn4
  Sensing i/RConn1 -- Meas P/LConn5
  Sensing i/RConn2 -- -/RConn1
  Motor/LConn2 -- +/RConn1
  Sensing i/LConn1 -- Motor/RConn3
  RevolutePivotBicep/LConn1 -- B/RConn1
  RevolutePivotBicep/RConn1 -- F/RConn1
  Motor/LConn1 -- RevolutePivotBicep/LConn2
  Motor/RConn2 -- Meas P/LConn2 -- RevolutePivotBicep/RConn3
  Meas P/LConn3 -- RevolutePivotBicep/RConn4
  Meas P/LConn1 -- Motor/RConn1 -- RevolutePivotBicep/RConn2

== system DCMotorLibrary/Detailed Model/Amplifier ==
  In1 : Inport
  Bias : Bias
  Gain : Gain  Gain=voltGain
  Saturation : Saturate  UpperLimit=5  LowerLimit=-5
  Out1 : Outport
  wires:
  Saturation/1 -> Gain/1
  Bias/1 -> Saturation/1
  In1/1 -> Bias/1
  Gain/1 -> Out1/1

== system DCMotorLibrary/Open Loop Interface/Serial Motor Interface ==
  command : Inport  OutDataTypeStr=uint8  SampleTime=1/10
  10-bit to Angle : demoLibrary/Utilities/10-bit to Angle  SystemSampleTime=-1  Latency=0  AutoFrameSizeCalculation=off
  Analog Input : instrumentlib/Serial Receive  ComPortMenu=<Please select a port...>  ComPort=COM5  ObjConstructor=serial('COM5');  Header=A  Terminator=NULL ('\0')  DataSize=1  DataType=uint16  EnableBlockingMode=off  ActionDataUnavailable=Output last received value  CustomValue=0  SampleTime=1/100
  Display : Display
  Display1 : Display
  PWM Output : instrumentlib/Serial Send  ComPortMenu=<Please select a port...>  ComPort=COM5  ObjConstructor=serial('COM5');  Terminator=<none>  EnableBlockingMode=on
  Serial Configuration1 : instrumentlib/Serial Configuration  Priority=-200000  ComPortMenu=<Please select a port...>  ComPort=COM5  ObjConstructor=serial('COM5');  BaudRate=9600  DataBits=8  Parity=none  StopBits=1  FlowControl=none  Timeout=10  ByteOrder=LittleEndian
  Angle : Outport
  wires:
  Analog Input/1 -> Display1/1, 10-bit to Angle/1
  Analog Input/2 -> Display/1
  command/1 -> PWM Output/1
  10-bit to Angle/1 -> Angle/1
